simulink model "ManipRoboticoRegolazioneSpazioOperativo"  (R2025b)
settings: Solver=VariableStepAuto  StartTime=0.0  StopTime=10  RelTol=1e-3
values from neighbouring files (symbols this model uses):
  Kd = [15; 15]    [main.m]
  Kp = [20; 20]    [main.m]
settings Model: Creator=arman  LastModifiedBy=arman

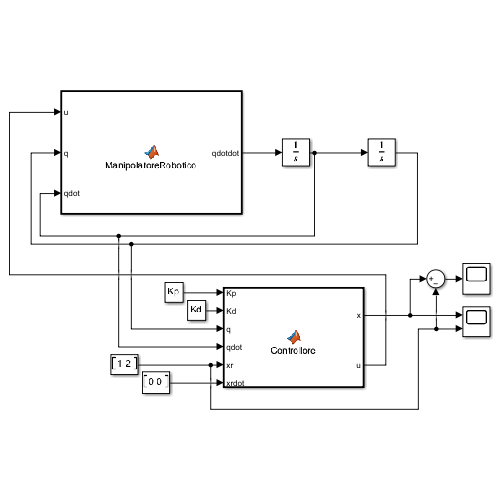
[thumbnail: Simulink's stored preview of the top-level diagram]
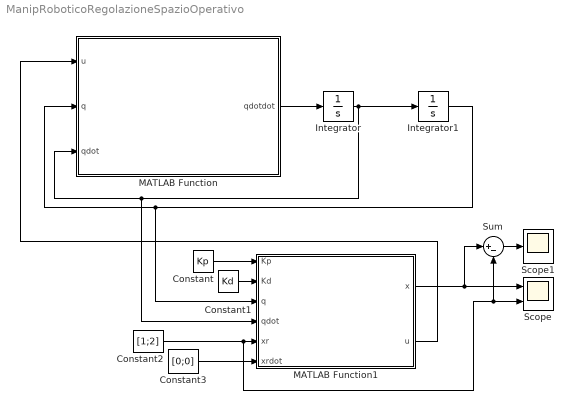
== system ManipRoboticoRegolazioneSpazioOperativo ==
  Constant : Constant  Value=Kp
  Constant1 : Constant  Value=Kd
  Constant2 : Constant  Value=[1;2]
  Constant3 : Constant  Value=[0;0]
  Integrator : Integrator  InitialCondition=[0;0]
  Integrator1 : Integrator  InitialCondition=[0;0]
  MATLAB Function : MATLAB Function  TreatAsAtomicUnit=on
  MATLAB Function1 : MATLAB Function  TreatAsAtomicUnit=on
  Scope : Scope  NumInputPorts=2
      settings: ActiveDisplayYMinimum=-0.71249999999999991  ActiveDisplayYMaximum=6.4125000000000005
  Scope1 : Scope
      settings: ActiveDisplayYMinimum=-2.8375  ActiveDisplayYMaximum=5.5375000000000005
  Sum : Sum  Inputs=|+-
  wires:
  Integrator/1 -> MATLAB Function/3(qdot), MATLAB Function1/4(qdot), Integrator1/1
  MATLAB Function/1(qdotdot) -> Integrator/1
  Integrator1/1 -> MATLAB Function1/3(q), MATLAB Function/2(q)
  MATLAB Function1/2(u) -> MATLAB Function/1(u)
  Constant/1 -> MATLAB Function1/1(Kp)
  Constant1/1 -> MATLAB Function1/2(Kd)
  Constant2/1 -> Sum/2, Scope/2, MATLAB Function1/5(xr)
  Constant3/1 -> MATLAB Function1/6(xrdot)
  MATLAB Function1/1(x) -> Sum/1, Scope/1
  Sum/1 -> Scope1/1

== matlab function ManipRoboticoRegolazioneSpazioOperativo/MATLAB Function1 ==
  data: x output; Kp input; u output; Kd input; q input; qdot input; xr input; xrdot input
function [x,u] = Controllore(Kp,Kd,q,qdot,xr,xrdot)

[B, C, g, F] = calculateMatrixRobotRR(q,qdot);

l1=3;
l2=2.7;
J = [-l1*sin(q(1))-l2*sin(q(1)+q(2))    -l2*sin(q(1)+q(2));
    l1*cos(q(1)) + l2*cos(q(1)+q(2))    l2*cos(q(1)+ q(2))];

x = [l1*cos(q(1)) + l2*cos(q(1)+q(2));
     l1*sin(q(1)) + l2*sin(q(1)+q(2))];
xdot = J * qdot;
e = x - xr;
edot = xdot - xrdot;
u = g - J.'*(Kd.*edot + Kp.*e);

== matlab function ManipRoboticoRegolazioneSpazioOperativo/MATLAB Function ==
  data: u input; qdotdot output; q input; qdot input
function qdotdot = ManipolatoreRobotico(u,q,qdot)
[B, C, g, F] = calculateMatrixRobotRR(q,qdot);
qdotdot = B \ (u - (C * qdot) - g - F);
